simulink model "control_model_gear_velocity"  (R2015a)
settings: Solver=ode45  StartTime=0  StopTime=10  FixedStep=0.01  RelTol=1e-3
libraries: simulink x1
settings Model: Creator=keysie  LastModifiedBy=keysie

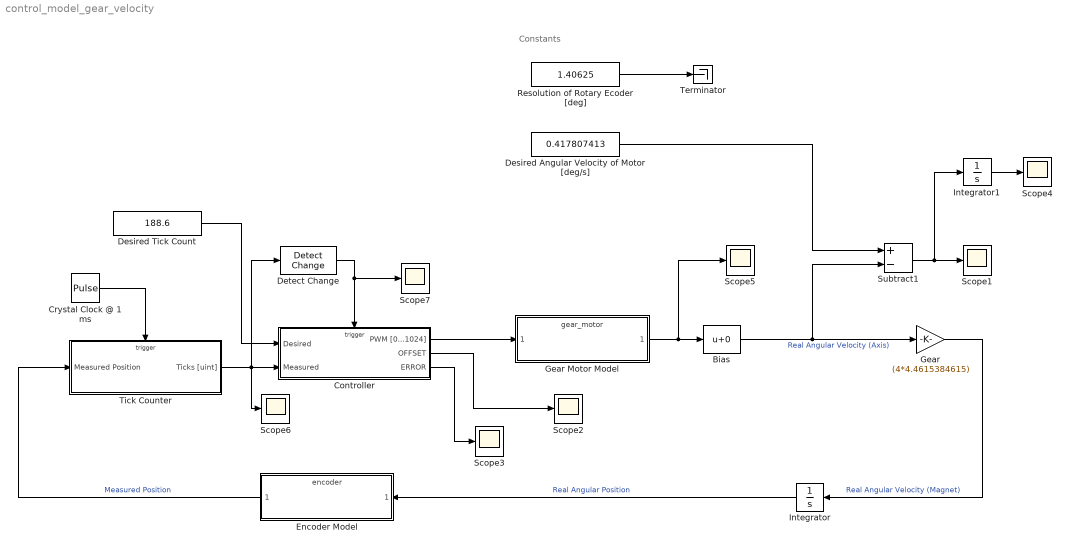
== system control_model_gear_velocity ==
  note: Constants
  Bias : Bias
  Controller : Subsystem  TreatAsAtomicUnit=on
  Crystal Clock @ 1 ms : DiscretePulseGenerator  PulseType=Time based  Period=0.001  PulseWidth=5
  Desired Angular Velocity of Motor [deg/s] : Constant  Value=0.417807413
  Desired Tick Count : Constant  Value=188.6
  Detect Change : simulink/Logic and Bit Operations/Detect Change  vinit=0  InputProcessing=Inherited  OutDataTypeStr=boolean
  Encoder Model : ModelReference  ModelNameDialog=encoder.slx  SimulationMode=Normal  ModelReferenceVersion=1.5  CopyOfModelName=encoder.slx  DefaultDataLogging=on
  Gear : Gain  Gain=(4*4.4615384615)
  Gear Motor Model : ModelReference  ModelNameDialog=gear_motor.slx  SimulationMode=Normal  ModelReferenceVersion=1.21  CopyOfModelName=gear_motor.slx  DefaultDataLogging=on
  Integrator : Integrator
  Integrator1 : Integrator
  Resolution of Rotary Ecoder [deg] : Constant  Value=1.40625
  Scope{1..7} (7 alike) : Scope
      Scope1 settings: TimeRange=300
      Scope2 settings: TimeRange=100  SaveName=ScopeData2
      Scope3 settings: SaveName=ScopeData6
      Scope4 settings: TimeRange=300
      Scope5 settings: TimeRange=300  SaveName=ScopeData3
      Scope6 settings: YMin=135000  YMax=170000  SaveName=ScopeData4
      Scope7 settings: YMin=135000  YMax=170000  SaveName=ScopeData5
  Subtract1 : Sum  Inputs=+-
  Terminator : Terminator
  Tick Counter : Subsystem  TreatAsAtomicUnit=on
  wires:
  Gear Motor Model/1 -> Scope5/1, Bias/1
  Integrator/1 -> Encoder Model/1  "Real Angular Position"
  Desired Tick Count/1 -> Controller/1(Desired)
  Controller/1(PWM [0...1024]) -> Gear Motor Model/1
  Controller/2(OFFSET) -> Scope2/1
  Subtract1/1 -> Integrator1/1, Scope1/1
  Controller/3(ERROR) -> Scope3/1
  Detect Change/1 -> Scope7/1, Controller/Trigger
  Desired Angular Velocity of Motor [deg/s]/1 -> Subtract1/1
  Resolution of Rotary Ecoder [deg]/1 -> Terminator/1
  Bias/1 -> Gear/1, Subtract1/2  "Real Angular Velocity (Axis)"
  Gear/1 -> Integrator/1  "Real Angular Velocity (Magnet)"
  Integrator1/1 -> Scope4/1
  Crystal Clock @ 1 ms/1 -> Tick Counter/Trigger
  Encoder Model/1 -> Tick Counter/1(Measured Position)  "Measured Position"
  Tick Counter/1(Ticks [uint]) -> Detect Change/1, Scope6/1, Controller/2(Measured)

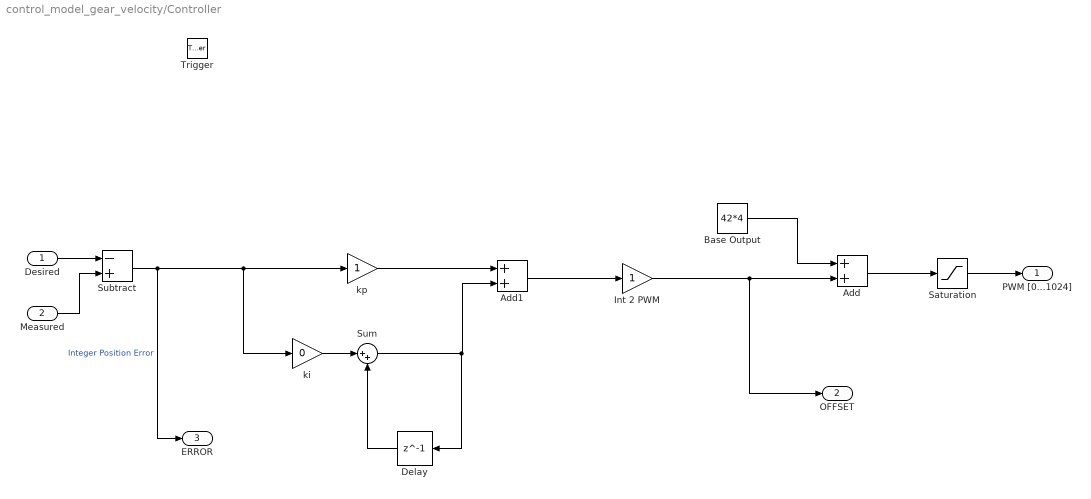
== system control_model_gear_velocity/Controller ==
  Desired : Inport
  Measured : Inport  Port=2
  Trigger : TriggerPort
  Add : Sum
  Add1 : Sum
  Base Output : Constant  Value=42*4
  Delay : Delay  DelayLength=1
  Int 2 PWM : Gain
  Saturation : Saturate  UpperLimit=1024  LowerLimit=0
  Subtract : Sum  Inputs=-+
  Sum : Sum  Inputs=|++
  ki : Gain  Gain=0
  kp : Gain
  PWM [0...1024] : Outport  InitialOutput=[0]
  OFFSET : Outport  Port=2  InitialOutput=[0]
  ERROR : Outport  Port=3  InitialOutput=[0]
  wires:
  Base Output/1 -> Add/1
  Add/1 -> Saturation/1
  Subtract/1 -> ERROR/1, ki/1, kp/1  "Integer Position Error"
  kp/1 -> Add1/1
  ki/1 -> Sum/1
  Add1/1 -> Int 2 PWM/1
  Int 2 PWM/1 -> OFFSET/1, Add/2
  Sum/1 -> Delay/1, Add1/2
  Delay/1 -> Sum/2
  Desired/1 -> Subtract/1
  Measured/1 -> Subtract/2
  Saturation/1 -> PWM [0...1024]/1

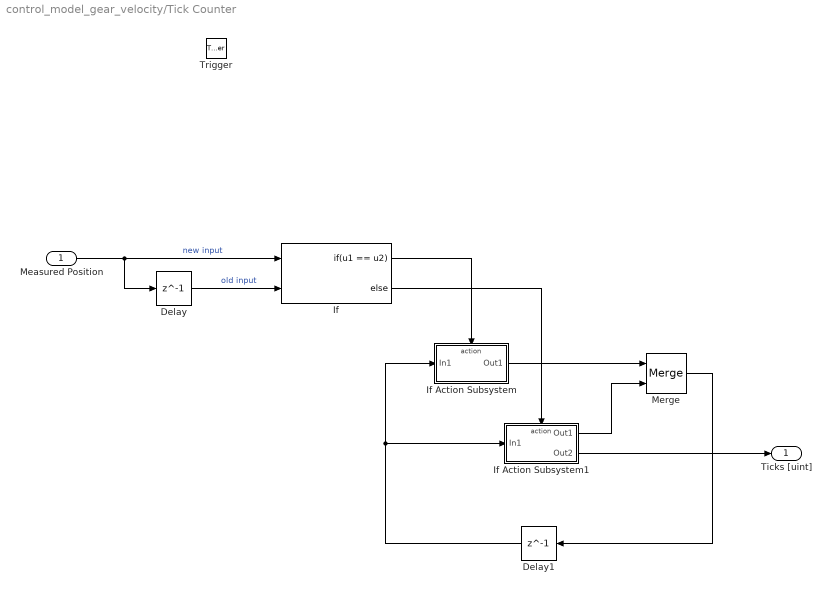
== system control_model_gear_velocity/Tick Counter ==
  Measured Position : Inport
  Trigger : TriggerPort
  Delay : Delay  DelayLength=1  InitialCondition=0
  Delay1 : Delay  DelayLength=1  InitialCondition=0
  If : If  NumInputs=2  IfExpression=u1 == u2
  If Action Subsystem : Subsystem  TreatAsAtomicUnit=on
  If Action Subsystem1 : Subsystem  TreatAsAtomicUnit=on
  Merge : Merge
  Ticks [uint] : Outport  InitialOutput=[0]
  wires:
  Measured Position/1 -> If/1, Delay/1  "new input"
  Delay/1 -> If/2  "old input"
  Merge/1 -> Delay1/1
  If/1 -> If Action Subsystem/Action
  If/2 -> If Action Subsystem1/Action
  If Action Subsystem/1(Out1) -> Merge/1
  If Action Subsystem1/1(Out1) -> Merge/2
  Delay1/1 -> If Action Subsystem1/1(In1), If Action Subsystem/1(In1)
  If Action Subsystem1/2(Out2) -> Ticks [uint]/1

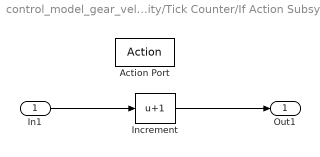
== system control_model_gear_velocity/Tick Counter/If Action Subsystem ==
  In1 : Inport
  Action Port : ActionPort  ActionType=then
  Increment : Bias  Bias=1
  Out1 : Outport  InitialOutput=0
  wires:
  In1/1 -> Increment/1
  Increment/1 -> Out1/1

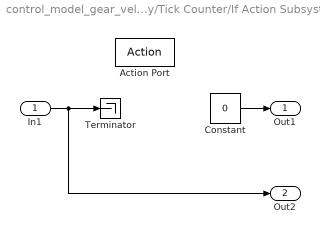
== system control_model_gear_velocity/Tick Counter/If Action Subsystem1 ==
  In1 : Inport
  Action Port : ActionPort  ActionType=else
  Constant : Constant  Value=0
  Terminator : Terminator
  Out1 : Outport  InitialOutput=0
  Out2 : Outport  Port=2  InitialOutput=0
  wires:
  Constant/1 -> Out1/1
  In1/1 -> Out2/1, Terminator/1
